simulink model "vision_processing"  (R2013a)
settings: Solver=FixedStepDiscrete  StartTime=0.0  StopTime=20.0  FixedStep=0.05  RelTol=1e-3
undefined symbols (not defined in the file): darwinop_communication_setup
libraries: simulink x4, lib_darwinop x1
settings Model: Creator=florent  LastModifiedBy=florent
settings OptimizationCC: OptimizeModelRefInitCode=on  LifeSpan=1
settings HardwareCC: ProdEndianess=LittleEndian  ProdHWDeviceType=Generic->32-bit Embedded Processor
settings RTWCC: SystemTargetFile=darwinoplib.tlc  TemplateMakefile=darwinoplib.tmf  Description=DarwinOP code generator  ProcessScript=darwinoplib_make_rtw_hook  TargetLang=C++
settings CodeAppCC: IgnoreCustomStorageClasses=off
settings STFCustomTargetCC: CombineOutputUpdateFcns=on  ERTCustomFileBanners=on  SupportContinuousTime=off  SupportNonInlinedSFcns=off  MATLABClassNameForMDSCustomization=Simulink.SoftwareTarget.ERTCustomization  SystemTargetFile=darwinoplib.tlc
settings ERTTargetCC: GenerateSampleERTMain=off  ParMdlRefBuildCompliant=off  CompOptLevelCompliant=off  ConcurrentExecutionCompliant=off  ERTFirstTimeCompliant=off  ModelStepFunctionPrototypeControlCompliant=off  CPPClassGenCompliant=off  ERTCustomFileTemplate=darwinoplib_main.tlc

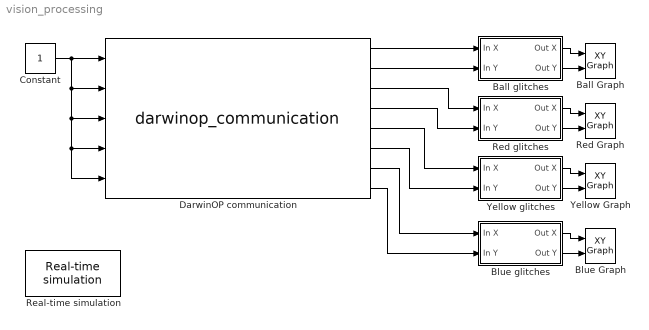
== system vision_processing ==
  Ball Graph : simulink/Sinks/XY Graph  xmin=0  xmax=320  ymin=0  ymax=240  st=-1
  Ball glitches : Subsystem
  Blue Graph : simulink/Sinks/XY Graph  xmin=0  xmax=320  ymin=0  ymax=240  st=-1
  Blue glitches : Subsystem
  Constant : Constant
  DarwinOP communication : M-S-Function  StartFcn=darwinop_communication_setup('StartFcn');  StopFcn=darwinop_communication_setup('StopFcn');  FunctionName=darwinop_communication  Parameters=IP,Port,Protocol,Timeout,Frame,ReadIndex,WriteIndex  mask{IP=192.168.123.1, Port=1234, Protocol=tcp, Timeout=0.05, Frame=[ 17 1 30 4 17 1 50 4 17 1 70 4 17 1 90 4 18 1 1 1 0 18 1 6 4 0 0 0 0], ReadIndex=[ 1 2;3 2;5 2;7 2;9 2;11 2;13 2;15 2], WriteIndex=[ 21 1;26 1;27 1;28 1;29 1]}
      settings: DeleteFcn=darwinop_communication_setup('DeleteFcn');  ModelCloseFcn=darwinop_communication_setup('ModelCloseFcn');  NameChangeFcn=darwinop_communication_setup('NameChangeFcn');  OpenFcn=darwinop_communication_setup('OpenFcn');
      mask TypeOptions Protocol: tcp | udp
      mask Display:
      | image('darwin-blk.jpg')
      | 
      | port_label('output',1,'Vision(1)/Ball X')
      | port_label('output',2,'Vision(1)/Ball Y')
      | port_label('output',3,'Vision(1)/Red X')
      | port_label('output',4,'Vision(1)/Red Y')
      | port_label('output',5,'Vision(1)/Yellow X')
      | port_label('output',6,'Vision(1)/Yellow Y')
      | port_label('output',7,'Vision(1)/Blue X')
      | port_label('output',8,'Vision(1)/Blue Y')
      | 
      | port_label('input',1,'Vision(1)/Enable')
      | port_label('input',2,'Vision(1)/Ball enable')
      | port_label('input',3,'Vision(1)/Red enable')
      | port_label('input',4,'Vision(1)/Yellow enable')
      | port_label('input',5,'Vision(1)/Blue enable')
  Real-time simulation : lib_darwinop/Real-time simulation  TimeScalingFactor=1
  Red Graph : simulink/Sinks/XY Graph  xmin=0  xmax=320  ymin=0  ymax=240  st=-1
  Red glitches : Subsystem
  Yellow Graph : simulink/Sinks/XY Graph  xmin=0  xmax=320  ymin=0  ymax=240  st=-1
  Yellow glitches : Subsystem
  wires:
  Constant/1 -> DarwinOP communication/5, DarwinOP communication/4, DarwinOP communication/3, DarwinOP communication/2, DarwinOP communication/1
  DarwinOP communication/1 -> Ball glitches/1(In X)
  Ball glitches/1(Out X) -> Ball Graph/1
  DarwinOP communication/2 -> Ball glitches/2(In Y)
  Ball glitches/2(Out Y) -> Ball Graph/2
  DarwinOP communication/3 -> Red glitches/1(In X)
  Red glitches/1(Out X) -> Red Graph/1
  DarwinOP communication/4 -> Red glitches/2(In Y)
  Red glitches/2(Out Y) -> Red Graph/2
  DarwinOP communication/5 -> Yellow glitches/1(In X)
  Yellow glitches/1(Out X) -> Yellow Graph/1
  DarwinOP communication/6 -> Yellow glitches/2(In Y)
  Yellow glitches/2(Out Y) -> Yellow Graph/2
  DarwinOP communication/7 -> Blue glitches/1(In X)
  Blue glitches/1(Out X) -> Blue Graph/1
  DarwinOP communication/8 -> Blue glitches/2(In Y)
  Blue glitches/2(Out Y) -> Blue Graph/2

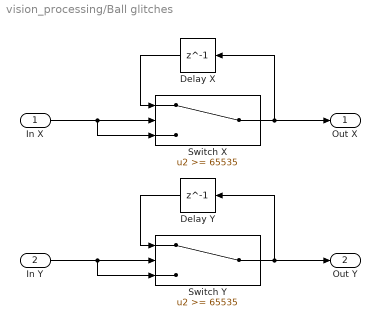
== system vision_processing/Ball glitches ==
  In X : Inport
  In Y : Inport  Port=2
  Delay X : Delay  DelayLength=1
  Delay Y : Delay  DelayLength=1
  Switch X : Switch  Threshold=65535
  Switch Y : Switch  Threshold=65535
  Out X : Outport
  Out Y : Outport  Port=2
  wires:
  Delay X/1 -> Switch X/1
  Switch X/1 -> Out X/1, Delay X/1
  In X/1 -> Switch X/3, Switch X/2
  Delay Y/1 -> Switch Y/1
  Switch Y/1 -> Out Y/1, Delay Y/1
  In Y/1 -> Switch Y/3, Switch Y/2

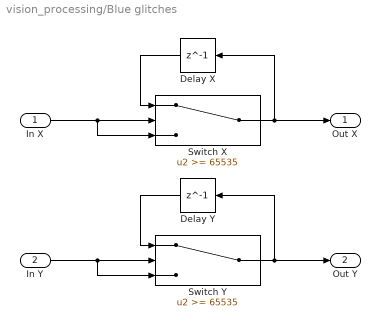
== system vision_processing/Blue glitches ==
  In X : Inport
  In Y : Inport  Port=2
  Delay X : Delay  DelayLength=1
  Delay Y : Delay  DelayLength=1
  Switch X : Switch  Threshold=65535
  Switch Y : Switch  Threshold=65535
  Out X : Outport
  Out Y : Outport  Port=2
  wires:
  Delay X/1 -> Switch X/1
  Switch X/1 -> Out X/1, Delay X/1
  In X/1 -> Switch X/3, Switch X/2
  Delay Y/1 -> Switch Y/1
  Switch Y/1 -> Out Y/1, Delay Y/1
  In Y/1 -> Switch Y/3, Switch Y/2

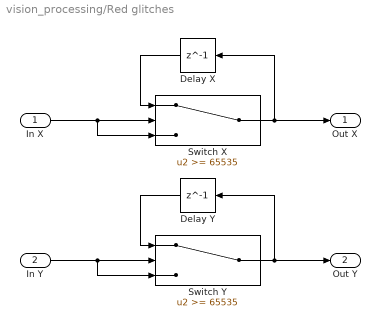
== system vision_processing/Red glitches ==
  In X : Inport
  In Y : Inport  Port=2
  Delay X : Delay  DelayLength=1
  Delay Y : Delay  DelayLength=1
  Switch X : Switch  Threshold=65535
  Switch Y : Switch  Threshold=65535
  Out X : Outport
  Out Y : Outport  Port=2
  wires:
  Delay X/1 -> Switch X/1
  Switch X/1 -> Out X/1, Delay X/1
  In X/1 -> Switch X/3, Switch X/2
  Delay Y/1 -> Switch Y/1
  Switch Y/1 -> Out Y/1, Delay Y/1
  In Y/1 -> Switch Y/3, Switch Y/2

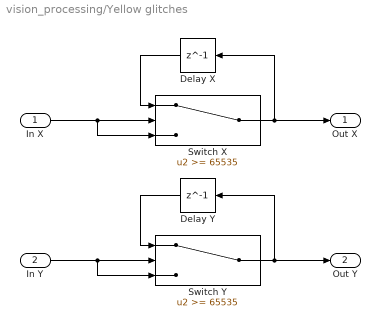
== system vision_processing/Yellow glitches ==
  In X : Inport
  In Y : Inport  Port=2
  Delay X : Delay  DelayLength=1
  Delay Y : Delay  DelayLength=1
  Switch X : Switch  Threshold=65535
  Switch Y : Switch  Threshold=65535
  Out X : Outport
  Out Y : Outport  Port=2
  wires:
  Delay X/1 -> Switch X/1
  Switch X/1 -> Out X/1, Delay X/1
  In X/1 -> Switch X/3, Switch X/2
  Delay Y/1 -> Switch Y/1
  Switch Y/1 -> Out Y/1, Delay Y/1
  In Y/1 -> Switch Y/3, Switch Y/2
